simulink model "Passive_Road_Profile_3"  (R2017b)
settings: Solver=VariableStepAuto  StartTime=0.0  StopTime=40  RelTol=1e-3
undefined symbols (not defined in the file): sigbuilder_block
settings Model: Creator=LENOVO  LastModifiedBy=LENOVO

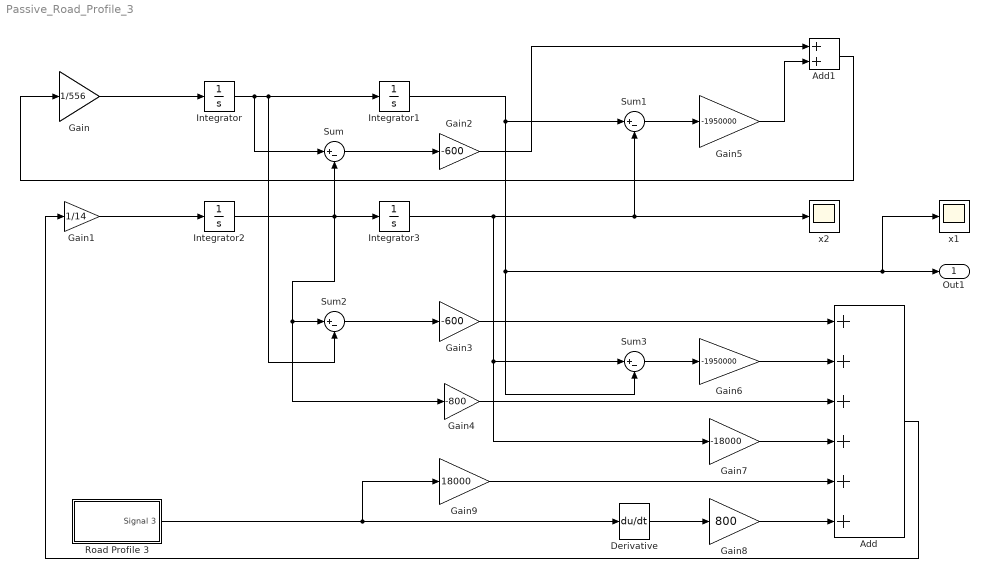
== system Passive_Road_Profile_3 ==
  Add : Sum  Inputs=++++++
  Add1 : Sum
  Derivative : Derivative
  Gain : Gain  Gain=1/556
  Gain1 : Gain  Gain=1/14
  Gain2 : Gain  Gain=-600
  Gain3 : Gain  Gain=-600
  Gain4 : Gain  Gain=-800
  Gain5 : Gain  Gain=-1950000
  Gain6 : Gain  Gain=-1950000
  Gain7 : Gain  Gain=-18000
  Gain8 : Gain  Gain=800
  Gain9 : Gain  Gain=18000
  Integrator{,1..3} (4 alike) : Integrator
  Road Profile 3 : Subsystem  Tag=STV Subsys  LoadFcn=sigbuilder_block('load');  StartFcn=sigbuilder_block('start');  StopFcn=sigbuilder_block('stop');  ClipboardFcn=sigbuilder_block('clipboard');  mask(Sigbuilder block){tuvar=[0:10]}
      mask help: Simulink:masks:SigbuilderBlock_MD
      mask init:
      | if ~strcmp(get_param(bdroot(gcbh),'SimulationStatus'),'stopped') tuvar = sigbuilder_block('maskInit'); end
      settings: CopyFcn=sigbuilder_block('copy');  DeleteFcn=sigbuilder_block('delete');  ModelCloseFcn=sigbuilder_block('modelClose');  PreSaveFcn=sigbuilder_block('preSave');  PauseFcn=sigbuilder_block('pause');  ContinueFcn=sigbuilder_block('continue');  NameChangeFcn=sigbuilder_block('namechange');  OpenFcn=sigbuilder_block('open',[141 130.5 550.5 359.25 ]);  CloseFcn=sigbuilder_block('close');
      mask Display: plot(0, 0, 100, 100,[2, 2, 32, 32, 2], [68, 8, 8, 68, 68],[32, 2], [38, 38], [32, 19, 2],[53, 60, 44], [32, 17, 17, 2],[16, 16, 31, 31]);txt = getActiveGroup(gcbh);text(2, 100, txt,'verticalAlignment', 'top');
  Sum{,1..3} (4 alike) : Sum  Inputs=|+-
  x1 : Scope
  x2 : Scope
  Out1 : Outport
  wires:
  Gain3/1 -> Add/1
  Gain4/1 -> Add/3
  Gain9/1 -> Add/5
  Gain7/1 -> Add/4
  Gain6/1 -> Add/2
  Gain8/1 -> Add/6
  Derivative/1 -> Gain8/1
  Road Profile 3/1(Signal 3) -> Derivative/1, Gain9/1
  Gain/1 -> Integrator/1
  Integrator/1 -> Sum/1, Sum2/2, Integrator1/1
  Gain5/1 -> Add1/2
  Sum/1 -> Gain2/1
  Gain2/1 -> Add1/1
  Sum1/1 -> Gain5/1
  Add1/1 -> Gain/1
  Gain1/1 -> Integrator2/1
  Integrator2/1 -> Sum2/1, Gain4/1, Sum/2, Integrator3/1
  Integrator3/1 -> Sum3/1, Gain7/1, Sum1/2, x2/1
  Sum2/1 -> Gain3/1
  Integrator1/1 -> Sum1/1, x1/1, Out1/1, Sum3/2
  Sum3/1 -> Gain6/1
  Add/1 -> Gain1/1

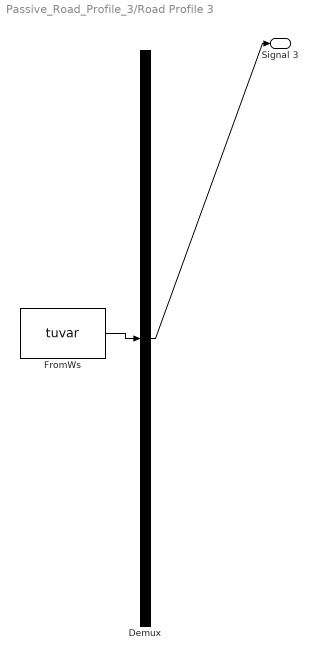
== system Passive_Road_Profile_3/Road Profile 3 ==
  Demux : Demux  Tag=STV Demux  Outputs=1
  FromWs : FromWorkspace  Tag=STV FromWs  VariableName=tuvar  SampleTime=0
      SigBuilderData=|
      | common.afterFinalStr = 'Extrapolate'
      | common.sampleTime = 0
      | dataSet.timeRange = [0 5]
      | dataSet.name = 'Group 1'
      | sbobj.Groups.Name = 'Group 1'
      | sbobj.Groups.Signals.Name = 'Signal 3'
      | sbobj.Groups.Signals.XData = [0 0.2 0.3 0.4 0.5 0.6 0.8 0.9 1 1.1 1.2 1.3 1.4 1.5 1.6 1.7 1.8 1.9 2 2.1 2.2 2.3 2.4 2.5 2.6 2.7 2.8 2.9 3 3.2 3.4 3.5 3.6 3.7 3.8 3.9 4 4.1 4.2 4.3 4.4 4.5 4.6 4.7 4.8 4.9 5]
      | sbobj.Groups.Signals.YData = [0 0 0 0 0 0.1 0 0 0 0 0 0 0 0 0 0 0 0 0 0 0 0 0 0 0 0 0 0 0 0.05 0 0 0 0 0 0 0 0 0 0 0 0 0 0 0 0 0]
      | sbobj.Groups.TimeRange = [0 5]
  Signal 3 : Outport  Tag=STV Outport
  wires:
  FromWs/1 -> Demux/1
  Demux/1 -> Signal 3/1
